simulink model "5MW_WIND_TURBINE_SCL_CONTROLLER_SIMULINK"  (R2025b)
settings: Solver=FixedStepAuto  StartTime=0.0  StopTime=TMax  FixedStep=0.0125  MaxStep=DT  RelTol=1e-3  EnableMultiTasking=on
PreLoadFcn:
  | Run_OpenFAST
undefined symbols (not defined in the file): OutList, strmatch, TMax
libraries: PLCSimAdvancedBlockLibrary x1
settings Model: Creator=bjonkman  LastModifiedBy=germa
settings SolverCC: AlgebraicLoopSolver=TrustRegion
settings DataIOCC: LimitDataPoints=on  SaveFormat=Array  SignalLoggingSaveFormat=ModelDataLogs  SaveOutput=off  SaveTime=off  ReturnWorkspaceOutputs=off  SignalLoggingName=sigsOut
settings OptimizationCC: ExpressionDepthLimit=2147483647.0  LifeSpan=inf
settings DebuggingCC: SaveWithParameterizedLinksMsg=none  UnderspecifiedInitializationDetection=Classic  MergeDetectMultiDrivingBlocksExec=none  SignalResolutionControl=TryResolveAllWithWarning  MultiTaskDSMMsg=warning  MultiTaskCondExecSysMsg=none  FcnCallInpInsideContextMsg=warning  UnconnectedInputMsg=warning  UnconnectedOutputMsg=warning  UnconnectedLineMsg=warning  StateNameClashWarn=warning  SFUnexpectedBacktrackingDiag=warning  SFNoUnconditionalDefaultTransitionDiag=warning  SFExecutionAtInitializationDiag=none  ArithmeticOperatorsInVariantConditions=warning
settings HardwareCC: ProdBitPerPointer=32.0  ProdBitPerSizeT=32.0  ProdBitPerPtrDiffT=32.0  ProdLargestAtomicFloat=None  ProdIntDivRoundTo=Undefined  ProdEndianess=Unspecified  ProdWordSize=32.0  ProdHWDeviceType=32-bit Generic  TargetUnknown=on
settings ModelReferenceCC: EnableRefExpFcnMdlSchedulingChecks=on  PropagateSignalLabelsOutOfModel=off
settings SFSimCC: SimUseLocalCustomCode=off  CustomCodeUndefinedFunction=UseInterfaceOnly
settings RTWCC: RTWUseLocalCustomCode=off  GPUComputeCapability=3.5  DLArmComputeVersion=19.05
settings CodeAppCC: StateflowObjectComments=on
settings GRTTargetCC: TargetLangStandard=C89/C90 (ANSI)  CombineOutputUpdateFcns=off  GRTInterface=on
settings ConfigComp: CovMetricSettings=dw  CovSaveCumulativeToWorkspaceVar=on  CovSaveSingleToWorkspaceVar=on  CovExternalEMLEnable=off

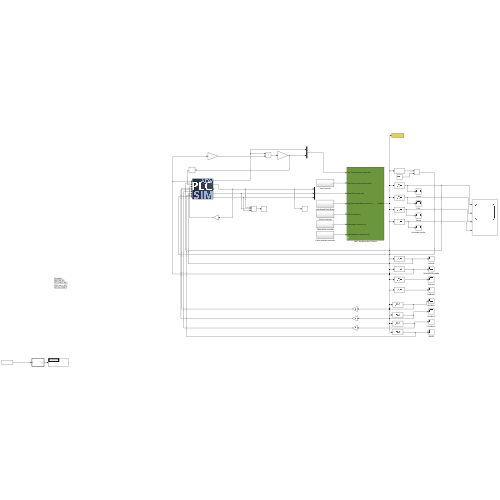
[thumbnail: Simulink's stored preview of the top-level diagram]
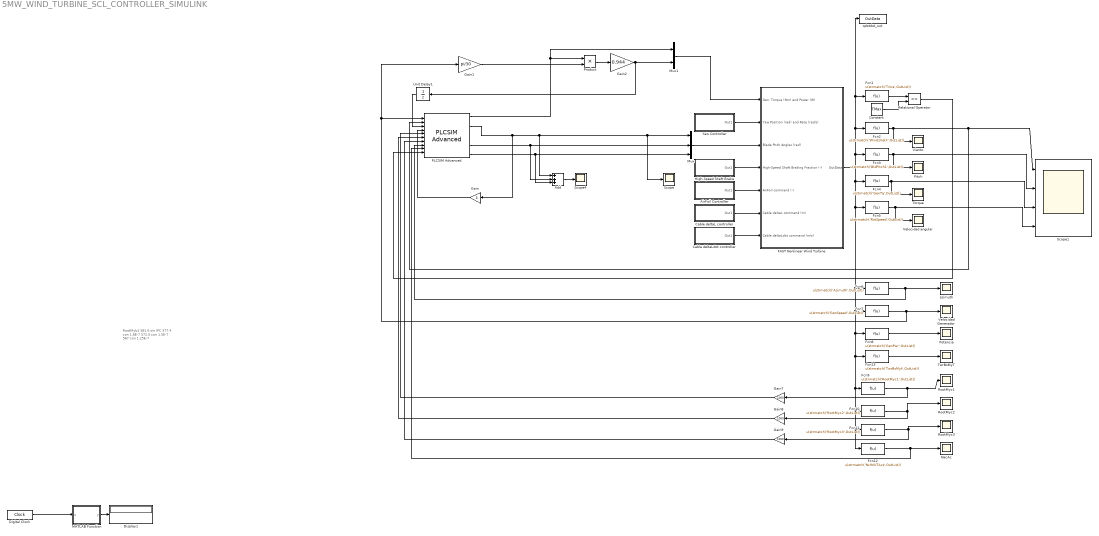
== system 5MW_WIND_TURBINE_SCL_CONTROLLER_SIMULINK ==
  note: RootMyb1
      | 581.6 sin IPC
      | 577.4 con 1.8E-7
      | 572.0 con 1.5E-7
      | 567 con 1.25E-7
  Add : Sum  Inputs=+++
  AirFoil Controller : Subsystem
  Cable deltaL controller : Subsystem
  Cable deltaLdot controller : Subsystem
  Constant : Constant  Value=TMax
  Digital Clock : DigitalClock
  Display1 : Display
  FAST Nonlinear Wind Turbine : Subsystem  mask(FAST Nonlinear Wind Turbine){}
      mask help: This block contains the FAST S-Function.
      mask init:
      | clear FAST_SFunc
  Fcn1 : Fcn  Expr=u(strmatch('Time',OutList))
  Fcn10 : Fcn  Expr=u(strmatch('RootMyc2',OutList))
  Fcn11 : Fcn  Expr=u(strmatch('RootMyc3',OutList))
  Fcn12 : Fcn  Expr=u(strmatch('NcIMUTAxs',OutList))
  Fcn13 : Fcn  Expr=u(strmatch('TwrBsMyt',OutList))
  Fcn2 : Fcn  Expr=u(strmatch('Wind1VelX',OutList))
  Fcn3 : Fcn  Expr=u(strmatch('BldPitch1',OutList))
  Fcn4 : Fcn  Expr=u(strmatch('GenTq',OutList))
  Fcn5 : Fcn  Expr=u(strmatch('RotSpeed',OutList))
  Fcn6 : Fcn  Expr=u(strmatch('Azimuth',OutList))
  Fcn7 : Fcn  Expr=u(strmatch('GenSpeed',OutList))
  Fcn8 : Fcn  Expr=u(strmatch('GenPwr',OutList))
  Fcn9 : Fcn  Expr=u(strmatch('RootMyc1',OutList))
  Gain : Gain
  Gain1 : Gain  Gain=pi/30
  Gain2 : Gain  Gain=0.944
  Gain7 : Gain  Gain=1000
  Gain8 : Gain  Gain=1000
  Gain9 : Gain  Gain=1000
  High-Speed Shaft Brake : Subsystem
  MATLAB Function : MATLAB Function  TreatAsAtomicUnit=on
  Mux : Mux  Inputs=3
  Mux1 : Mux  Inputs=2
  NacAc : Scope
      settings: ActiveDisplayYMinimum=-0.83860660344362259  ActiveDisplayYMaximum=0.69692713767290115  DataLoggingVariableName=ScopeData14
  PLCSIM Advanced : PLCSimAdvancedBlockLibrary/PLCSIM Advanced  Description=PLCSim Advanced S-Function  InstanceName='Turbina_5MW_NREL'  ScaleFactor=1  InputPortCount=10  OutputPortCount=5  InputVariables=''  OutputVariables=''  Synchronization=on  PIP=0  Networking=off  IP='localhost'  Port=4567  SampleTime=-1
  Pitch : Scope
      settings: ActiveDisplayYMinimum=-2.4085474386811252  ActiveDisplayYMaximum=16.520306803286076
  Potencia : Scope
      settings: ActiveDisplayYMinimum=4740.8865088226139  ActiveDisplayYMaximum=5230.1662979125413  DataLoggingVariableName=ScopeData6
  Product : Product
  Relational Operator : RelationalOperator  Operator===  OutDataTypeStr=boolean  RndMeth=Simplest  InputSameDT=off
  RootMyc1 : Scope
      settings: ActiveDisplayYMinimum=-3235.3011169433594  ActiveDisplayYMaximum=13706.296478271484  DataLoggingVariableName=ScopeData10
  RootMyc2 : Scope
      settings: ActiveDisplayYMinimum=-1293.7149896621702  ActiveDisplayYMaximum=12203.355484962463  DataLoggingVariableName=ScopeData11
  RootMyc3 : Scope
      settings: ActiveDisplayYMinimum=-7269.1810302734375  ActiveDisplayYMaximum=13276.730834960938  DataLoggingVariableName=ScopeData12
  Scope : Scope
      settings: ActiveDisplayYMinimum=-0.036474950262345367  ActiveDisplayYMaximum=0.29579697793815285  DataLoggingVariableName=ScopeData4
  Scope1 : Scope  NumInputPorts=4
      settings: ActiveDisplayString=3  Title=Par electromagnético (kNm)  ActiveDisplayYMinimum=2.0957872867584237  ActiveDisplayYMaximum=52.474031209945679  DataLoggingVariableName=ScopeData9
  Scope4 : Scope
      settings: ActiveDisplayYMinimum=-0.037476172670722  ActiveDisplayYMaximum=0.33728555403649807  DataLoggingVariableName=ScopeData16
  Torque : Scope
      settings: ActiveDisplayYMinimum=6.2351031899452209  ActiveDisplayYMaximum=6.5486707091331482  DataLoggingVariableName=ScopeData2
  TwrBsMyT : Scope
      settings: ActiveDisplayYMinimum=-84399.39990234375  ActiveDisplayYMaximum=118889.16943359375  DataLoggingVariableName=ScopeData15
  Unit Delay1 : UnitDelay  SampleTime=-1  HasFrameUpgradeWarning=on
  Velocidad Generador : Scope
      settings: ActiveDisplayYMinimum=340.67295970651367  ActiveDisplayYMaximum=1898.4378386032547  DataLoggingVariableName=ScopeData7
  Velocidad angular : Scope
      settings: ActiveDisplayYMinimum=-9.0503578404682656  ActiveDisplayYMaximum=25.967705687566145  DataLoggingVariableName=ScopeData3
  Viento : Scope
      settings: ActiveDisplayYMinimum=8.9999988079071045  ActiveDisplayYMaximum=9.0000011920928955
  Yaw Controller : Subsystem
  azimuth : Scope
      settings: ActiveDisplayYMinimum=-44.970661163330071  ActiveDisplayYMaximum=404.7359504699707  DataLoggingVariableName=ScopeData13
  qdotdot_out : ToWorkspace  VariableName=OutData  SampleTime=-1
  wires:
  FAST Nonlinear Wind Turbine/1(OutData) -> Fcn3/1, Fcn2/1, qdotdot_out/1, Fcn1/1, Fcn5/1, Fcn7/1, Fcn8/1, Fcn13/1, Fcn9/1, Fcn10/1, Fcn11/1, Fcn12/1, Fcn6/1, Fcn4/1
  Yaw Controller/1(Out1) -> FAST Nonlinear Wind Turbine/2(Yaw Position (rad) and Rate (rad/s))
  High-Speed Shaft Brake/1(Out1) -> FAST Nonlinear Wind Turbine/4(High-Speed Shaft Braking Fraction (-))
  AirFoil Controller/1(Out1) -> FAST Nonlinear Wind Turbine/5(AirFoil command (-))
  Cable deltaL controller/1(Out1) -> FAST Nonlinear Wind Turbine/6(Cable deltaL command (m))
  Cable deltaLdot controller/1(Out1) -> FAST Nonlinear Wind Turbine/7(Cable deltaLdot command (m/s))
  Fcn3/1 -> Pitch/1, Scope1/2
  Fcn4/1 -> Torque/1, Scope1/3
  Mux/1 -> FAST Nonlinear Wind Turbine/3(Blade Pitch Angles (rad))
  Mux1/1 -> FAST Nonlinear Wind Turbine/1(Gen. Torque (Nm) and Power (W))
  Fcn5/1 -> Velocidad angular/1, Scope1/4
  Fcn8/1 -> Potencia/1
  Product/1 -> Gain2/1
  Gain1/1 -> Product/2
  PLCSIM Advanced/1 -> Mux1/1, Product/1
  Digital Clock/1 -> MATLAB Function/1(u)
  MATLAB Function/1(y) -> Display1/1
  PLCSIM Advanced/2 -> Gain/1, Scope/1, Mux/1, Add/1
  Fcn7/1 -> Gain1/1, PLCSIM Advanced/1, Velocidad Generador/1
  Fcn2/1 -> Viento/1, PLCSIM Advanced/2, Scope1/1
  Gain2/1 -> Unit Delay1/1, Mux1/2
  Fcn9/1 -> RootMyc1/1, Gain7/1
  Fcn10/1 -> RootMyc2/1, Gain8/1
  Fcn11/1 -> RootMyc3/1, Gain9/1
  Fcn6/1 -> PLCSIM Advanced/8, azimuth/1
  Unit Delay1/1 -> PLCSIM Advanced/3
  Fcn12/1 -> PLCSIM Advanced/9, NacAc/1
  Fcn13/1 -> TwrBsMyT/1
  Constant/1 -> Relational Operator/2
  Relational Operator/1 -> PLCSIM Advanced/10
  Gain7/1 -> PLCSIM Advanced/5
  Gain8/1 -> PLCSIM Advanced/6
  Gain9/1 -> PLCSIM Advanced/7
  Add/1 -> Scope4/1
  PLCSIM Advanced/4 -> Mux/2, Add/2
  PLCSIM Advanced/5 -> Mux/3, Add/3
  Fcn1/1 -> Relational Operator/1
  Gain/1 -> PLCSIM Advanced/4

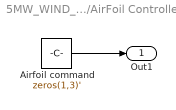
== system 5MW_WIND_TURBINE_SCL_CONTROLLER_SIMULINK/AirFoil Controller ==
  Airfoil command : Constant  Value=zeros(1,3)'
  Out1 : Outport
  wires:
  Airfoil command/1 -> Out1/1

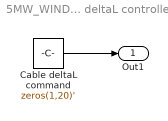
== system 5MW_WIND_TURBINE_SCL_CONTROLLER_SIMULINK/Cable deltaL controller ==
  Cable deltaL command : Constant  Value=zeros(1,20)'
  Out1 : Outport
  wires:
  Cable deltaL command/1 -> Out1/1

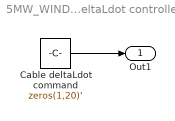
== system 5MW_WIND_TURBINE_SCL_CONTROLLER_SIMULINK/Cable deltaLdot controller ==
  Cable deltaLdot command : Constant  Value=zeros(1,20)'
  Out1 : Outport
  wires:
  Cable deltaLdot command/1 -> Out1/1

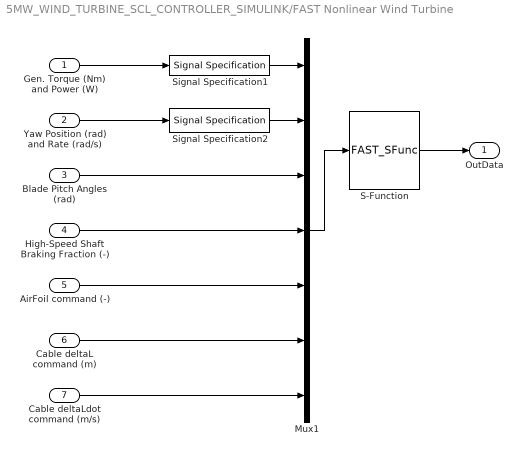
== system 5MW_WIND_TURBINE_SCL_CONTROLLER_SIMULINK/FAST Nonlinear Wind Turbine ==
  Gen. Torque (Nm) and Power (W) : Inport
  Yaw Position (rad) and Rate (rad/s) : Inport  Port=2
  Blade Pitch Angles (rad) : Inport  Port=3
  High-Speed Shaft Braking Fraction (-) : Inport  Port=4
  AirFoil command (-) : Inport  Port=5
  Cable deltaL command (m) : Inport  Port=6
  Cable deltaLdot command (m/s) : Inport  Port=7
  Mux1 : Mux  Inputs=7
  S-Function : S-Function  FunctionName=FAST_SFunc  Parameters=FAST_InputFileName, TMax, 0  SFunctionDeploymentMode=off  EnableBusSupport=off
  Signal Specification1 : SignalSpecification  OutDataTypeStr=double  Dimensions=2
  Signal Specification2 : SignalSpecification  OutDataTypeStr=double  Dimensions=2
  OutData : Outport
  wires:
  Gen. Torque (Nm) and Power (W)/1 -> Signal Specification1/1
  S-Function/1 -> OutData/1
  Mux1/1 -> S-Function/1
  Blade Pitch Angles (rad)/1 -> Mux1/3
  Yaw Position (rad) and Rate (rad/s)/1 -> Signal Specification2/1
  Signal Specification1/1 -> Mux1/1
  Signal Specification2/1 -> Mux1/2
  High-Speed Shaft Braking Fraction (-)/1 -> Mux1/4
  AirFoil command (-)/1 -> Mux1/5
  Cable deltaL command (m)/1 -> Mux1/6
  Cable deltaLdot command (m/s)/1 -> Mux1/7

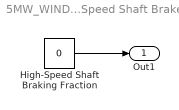
== system 5MW_WIND_TURBINE_SCL_CONTROLLER_SIMULINK/High-Speed Shaft Brake ==
  High-Speed Shaft Braking Fraction : Constant  Value=0
  Out1 : Outport
  wires:
  High-Speed Shaft Braking Fraction/1 -> Out1/1

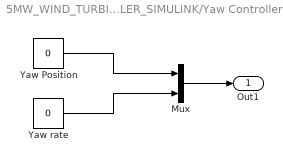
== system 5MW_WIND_TURBINE_SCL_CONTROLLER_SIMULINK/Yaw Controller ==
  Mux : Mux  Inputs=2
  Yaw Position : Constant  Value=0
  Yaw rate : Constant  Value=0
  Out1 : Outport
  wires:
  Mux/1 -> Out1/1
  Yaw Position/1 -> Mux/1
  Yaw rate/1 -> Mux/2

== matlab function 5MW_WIND_TURBINE_SCL_CONTROLLER_SIMULINK/MATLAB Function ==
  data: u input; y output
function y = fcn(u)
    minutos = floor(u/60);
    segundos = mod(u,60);
    % Esto devuelve un vector o puedes usar sprintf para strings
    y = [minutos; segundos]; 
end
